simulink model "MDCC_DeadComp"  (R2023a)
settings: Solver=FixedStepDiscrete  StartTime=0.0  StopTime=10.0  FixedStep=0.0001  RelTol=1e-3
model workspace (MATLAB code in the model file):
  | cmdLim = Simulink.Parameter;
  | cmdLim.Value = 15;
  | cmdLim.Description = 'Limit for controlling the maximum surface command angle.';
  | cmdLim.Min = 0;
  | cmdLim.Max = 90;
  | cmdLim.DocUnits = 'deg';
  | 
  | dispGain = Simulink.Parameter;
  | dispGain.Value = 0.75;
  | dispGain.Description = 'Gain applied to the displacement error.';
  | dispGain.Min = 0;
  | dispGain.Max = [];
  | dispGain.DocUnits = 'deg/sec/deg';
  | 
  | dispLim = Simulink.Parameter;
  | dispLim.Value = 30;
  | dispLim.Description = 'Limit for controlling the maximum commanded angle.';
  | dispLim.Min = 0;
  | dispLim.Max = 180;
  | dispLim.DocUnits = 'deg';
  | 
  | intGain = Simulink.Parameter;
  | intGain.Value = 0.5;
  | intGain.Description = 'Gain applied to the integral error.';
  | intGain.Min = 0;
  | intGain.Max = [];
  | intGain.DocUnits = 'deg/sec/deg/sec';
  | 
  | intLim = Simulink.Parameter;
  | intLim.Value = 5;
  | intLim.Description = 'Limit for controlling the maximum commanded angle.';
  | intLim.Min = 0;
  | intLim.Max = 90;
  | intLim.DocUnits = 'deg';
  | 
  | rateGain = Simulink.Parameter;
  | rateGain.Value = 2;
  | rateGain.Description = 'Gain applied to the rate error.';
  | rateGain.Min = 0;
  | rateGain.Max = [];
  | rateGain.DocUnits = 'deg/deg/sec';
  | 
  | rateLim = Simulink.Parameter;
  | rateLim.Value = 6;
  | rateLim.Description = 'Limit for controlling the maximum commanded angle.';
  | rateLim.Min = 0;
  | rateLim.Max = 180;
  | rateLim.DocUnits = 'deg/sec';
  | 
  | hdgGain = Simulink.Parameter;
  | hdgGain.Value = 0.015;
values from neighbouring files (symbols this model uses):
  Ts = 5E-6    (= 5e-06)    [iPMSM_data.m]
undefined symbols (not defined in the file or in its folder): CosTable12bit_Y, GLBCal_GLBCal_Kf_DCLinkOverVolErrThd_V, GLBCal_GLBCal_Kf_DCLinkUnderVolErrThd_V, GLBCal_GLBCal_Kf_EquiLd_NULL, GLBCal_GLBCal_Kf_EquiLq_NULL, GLBCal_GLBCal_Kf_MotorRatedSpeed_rpm, GLBCal_GLBCal_Kf_MotorSpeedHysteresis_Coef, GLBCal_Ke_MotorPolePairsNum_NULL, IoHwAbOpArg_PwmDutyCyclePhU_NULL, IoHwAbOpArg_PwmDutyCyclePhV_NULL, IoHwAbOpArg_PwmDutyCyclePhW_NULL, IoHwAbOpArg_PwmOutputEn, KbMDCC_DeadTimeCompEn_flg, KbMDCC_MCF_flgHarmInject_flg, KbMDCC_SetEAngleEn_flg, KbMDCC_UdUqFwOmit_flg, KfMDCC_AbsIs_A, KfMDCC_ActiveDischargeIdCurVal_A, KfMDCC_ActiveDischargeIqCurVal_A, KfMDCC_DCLinkVolRate_coef, KfMDCC_DeadRate_NULL, KfMDCC_DebugEAngleInit_rad, KfMDCC_DebugUalphaVolCmd_V, KfMDCC_DebugUbetaVolCmd_V, KfMDCC_DebugUdCmd_V, KfMDCC_DebugUqCmd_V, KfMDCC_DebugUsCmd_V, KfMDCC_DebugUsRate_V, KfMDCC_Duty_Coef, KfMDCC_IMCResp_NULL, KfMDCC_IMCStab_NULL, KfMDCC_InvParkCpPeriodTimesT_NULL, KfMDCC_MCF_Harm1113FLParamSpeedThrd_rads, KfMDCC_MCF_Harm57FLParamSpeedThrd_rads, KfMDCC_MCF_HarmCpnAg_NULL, KfMDCC_MCF_HarmfLParaHigh_coef, KfMDCC_MCF_HarmfLParaLow_coef, KfMDCC_MCF_HarmInSpdLimt_rpm, KfMDCC_MCF_HarmInUAlphaMax_V, KfMDCC_MCF_HarmInUbetaMax_V, KfMDCC_MotorSpeedRadsDAQFactor_NULL, KfMDCC_ResScal_Coef, KfMDCC_SelfHeatingUdVal_V, KfMDCC_SelfHeatingUdValRate_V, KfMDCC_SpdIMCResp_rpm, KfMDCC_SpdIMCStab_rpm, KfMDCC_VfMDCC_DCLinkCurValFactor_NULL, KfMDCM_DCLinkCoef, KfMDCM_DCLinkRatedVoltage_V, KfMDCM_FluxWeakningVolFWOffset_V, KuMDCC_PositionResolution_NULL, KuMDCC_SetEAngle_Null, MDSM_MCUStatus, PiIoHwSetInvState_C_Sws_UVW_PwmEnOutput, PiIoHwSetInvState_C_SwsSet_DPO_UVW_Asc, PiIoHwSetInvState_C_SwsSet_DPO_UVW_FW, PiIoHwSetPwmDuty_C_SwsSet_DPO_UVW_Duty, SinTable12bit_Y, SVPWM, VfMDCC_DeadComSpeedHigh_Rpm ... (+5)
libraries: simulink x14, PMSM_Library x4
(part 3 of 6)

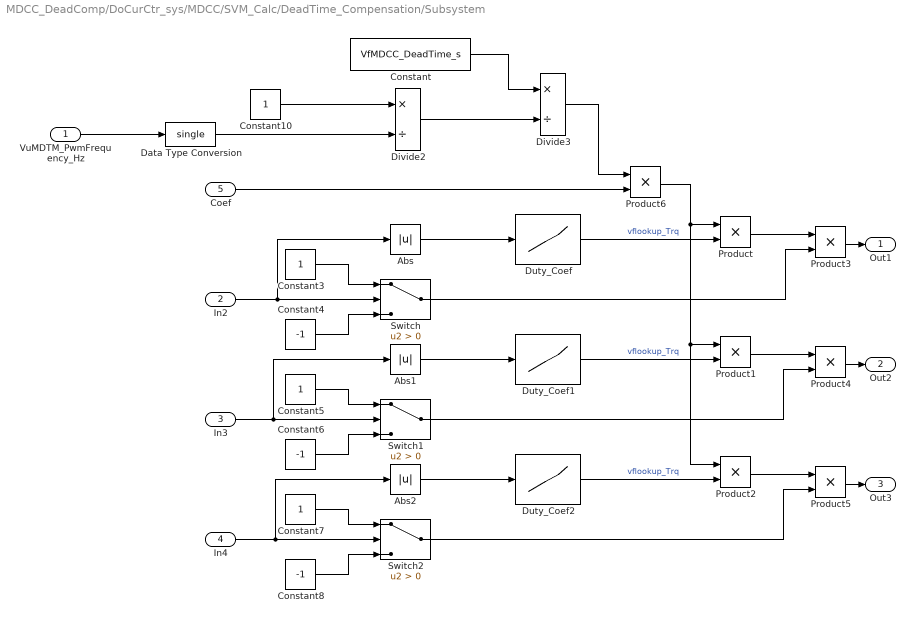
== system MDCC_DeadComp/DoCurCtr_sys/MDCC/SVM_Calc/DeadTime_Compensation/Subsystem ==
  VuMDTM_PwmFrequency_Hz : Inport
  In2 : Inport  Port=2
  In3 : Inport  Port=3
  In4 : Inport  Port=4
  Coef : Inport  Port=5
  Abs : Abs  SaturateOnIntegerOverflow=off
  Abs1 : Abs  SaturateOnIntegerOverflow=off
  Abs2 : Abs  SaturateOnIntegerOverflow=off
  Constant : Constant  Value=VfMDCC_DeadTime_s  OutDataTypeStr=single
  Constant10 : Constant  OutDataTypeStr=single
  Constant3 : Constant  OutDataTypeStr=int8
  Constant4 : Constant  Value=-1  OutDataTypeStr=int8
  Constant5 : Constant  OutDataTypeStr=int8
  Constant6 : Constant  Value=-1  OutDataTypeStr=int8
  Constant7 : Constant  OutDataTypeStr=int8
  Constant8 : Constant  Value=-1  OutDataTypeStr=int8
  Data Type Conversion : DataTypeConversion  OutDataTypeStr=single  SaturateOnIntegerOverflow=off  RndMeth=Floor
  Divide2 : Product  Inputs=*/
  Divide3 : Product  Inputs=*/
  Duty_Coef : Lookup_n-D  NumberOfTableDimensions=1  BreakpointsForDimension1=KfMDCC_AbsIs_A  BreakpointsForDimension1DataTypeStr=Inherit: Inherit from 'Breakpoint data'  IndexSearchMethod=Linear search  Table=KfMDCC_Duty_Coef  TableDataTypeStr=Inherit: Inherit from 'Table data'  ExtrapMethod=Clip  UseLastTableValue=on  InternalRulePriority=Speed  OutDataTypeStr=Inherit: Inherit from 'Table data'  RndMeth=Simplest  InputSameDT=off
  Duty_Coef1 : Lookup_n-D  NumberOfTableDimensions=1  BreakpointsForDimension1=KfMDCC_AbsIs_A  BreakpointsForDimension1DataTypeStr=Inherit: Inherit from 'Breakpoint data'  IndexSearchMethod=Linear search  Table=KfMDCC_Duty_Coef  TableDataTypeStr=Inherit: Inherit from 'Table data'  ExtrapMethod=Clip  UseLastTableValue=on  InternalRulePriority=Speed  OutDataTypeStr=Inherit: Inherit from 'Table data'  RndMeth=Simplest  InputSameDT=off
  Duty_Coef2 : Lookup_n-D  NumberOfTableDimensions=1  BreakpointsForDimension1=KfMDCC_AbsIs_A  BreakpointsForDimension1DataTypeStr=Inherit: Inherit from 'Breakpoint data'  IndexSearchMethod=Linear search  Table=KfMDCC_Duty_Coef  TableDataTypeStr=Inherit: Inherit from 'Table data'  ExtrapMethod=Clip  UseLastTableValue=on  InternalRulePriority=Speed  OutDataTypeStr=Inherit: Inherit from 'Table data'  RndMeth=Simplest  InputSameDT=off
  Product{,1..6} (7 alike) : Product
  Switch : Switch  Criteria=u2 > Threshold  SaturateOnIntegerOverflow=off  InputSameDT=off
  Switch1 : Switch  Criteria=u2 > Threshold  SaturateOnIntegerOverflow=off  InputSameDT=off
  Switch2 : Switch  Criteria=u2 > Threshold  SaturateOnIntegerOverflow=off  InputSameDT=off
  Out1 : Outport
  Out2 : Outport  Port=2
  Out3 : Outport  Port=3
  wires:
  Product/1 -> Product3/1
  Constant3/1 -> Switch/1
  Constant6/1 -> Switch1/3
  Constant8/1 -> Switch2/3
  Switch2/1 -> Product5/2
  Constant5/1 -> Switch1/1
  Duty_Coef1/1 -> Product1/2  "vflookup_Trq"
  Switch1/1 -> Product4/2
  Constant4/1 -> Switch/3
  Abs1/1 -> Duty_Coef1/1
  In4/1 -> Abs2/1, Switch2/2
  Product1/1 -> Product4/1
  Product2/1 -> Product5/1
  In3/1 -> Abs1/1, Switch1/2
  Constant7/1 -> Switch2/1
  Constant10/1 -> Divide2/1
  Abs2/1 -> Duty_Coef2/1
  Product5/1 -> Out3/1
  In2/1 -> Abs/1, Switch/2
  Duty_Coef2/1 -> Product2/2  "vflookup_Trq"
  Divide2/1 -> Divide3/2
  Duty_Coef/1 -> Product/2  "vflookup_Trq"
  Abs/1 -> Duty_Coef/1
  Constant/1 -> Divide3/1
  Switch/1 -> Product3/2
  Product3/1 -> Out1/1
  Product4/1 -> Out2/1
  VuMDTM_PwmFrequency_Hz/1 -> Data Type Conversion/1
  Data Type Conversion/1 -> Divide2/2
  Divide3/1 -> Product6/1
  Product6/1 -> Product2/1, Product1/1, Product/1
  Coef/1 -> Product6/2

== system MDCC_DeadComp/DoCurCtr_sys/MDCC/SVM_Calc/DeadTime_Compensation/TorqueDamping ==
  set : Inport
  Constant2 : Constant  Value=KfMDCC_DeadRate_NULL
  Delay : Delay  DelayLength=1
  Subsystem1 : Subsystem
  VfMDTL_TorqueCmd_Nm : Outport
  wires:
  Delay/1 -> Subsystem1/3(this_ref)
  Subsystem1/1(Out1) -> VfMDTL_TorqueCmd_Nm/1, Delay/1
  Constant2/1 -> Subsystem1/2(rate)
  set/1 -> Subsystem1/1(set)

== system MDCC_DeadComp/DoCurCtr_sys/MDCC/SVM_Calc/MDSA/SVPWM1 ==
  Ualpha_V : Inport
  Ubeta_V : Inport  Port=2
  Ts : Inport  Port=3
  Vdc : Inport  Port=4
  Bus Creator : BusCreator  Inputs=2
  Bus Creator1 : BusCreator  Inputs=2
  Bus Selector : BusSelector  OutputSignals=signal1,signal2,signal3
  Terminator : Terminator
  vIntp_PWMFOC_CalSec : Subsystem  TreatAsAtomicUnit=on  RTWFcnName=vIntp_PWMFOC_CalSec  RTWFileName=vIntp_PWMFOC_CalSec
      settings: RTWFcnNameOpts=User specified  RTWFileNameOpts=User specified
  vIntp_PWMFOC_CalTriCompValue : Subsystem  TreatAsAtomicUnit=on  RTWFcnName=vIntp_PWMFOC_CalTriCompValue  RTWFileName=vIntp_PWMFOC_CalTriCompValue
      settings: RTWFcnNameOpts=User specified  RTWFileNameOpts=User specified
  VfMDSA_PwmDutyCyclePhaseU_NULL : Outport
  VfMDSA_PwmDutyCyclePhaseV_NULL : Outport  Port=2
  VfMDSA_PwmDutyCyclePhaseW_NULL : Outport  Port=3
  wires:
  Bus Creator1/1 -> vIntp_PWMFOC_CalTriCompValue/3(Bus_Ts_Vdc)
  Vdc/1 -> Bus Creator1/2  "Vdc"
  Ts/1 -> Bus Creator1/1  "Ts"
  Ubeta_V/1 -> Bus Creator/2  "Ubeta"
  Ualpha_V/1 -> Bus Creator/1  "Ualpha"
  Bus Creator/1 -> vIntp_PWMFOC_CalSec/1(Bus_UalphaUbeta), vIntp_PWMFOC_CalTriCompValue/2(Bus_UalphaUbeta)
  vIntp_PWMFOC_CalSec/1(SecValue) -> Terminator/1
  vIntp_PWMFOC_CalSec/2(N_VALUE) -> vIntp_PWMFOC_CalTriCompValue/1(N_VALUE_IN)
  vIntp_PWMFOC_CalTriCompValue/1(Bus_CMP) -> Bus Selector/1
  Bus Selector/1 -> VfMDSA_PwmDutyCyclePhaseU_NULL/1  "<signal1>"
  Bus Selector/2 -> VfMDSA_PwmDutyCyclePhaseV_NULL/1  "<signal2>"
  Bus Selector/3 -> VfMDSA_PwmDutyCyclePhaseW_NULL/1  "<signal3>"

== system MDCC_DeadComp/DoCurCtr_sys/MDCC/SVM_Calc/MDSA/SVPWM_E ==
  Vsalfak : Inport
  Vsbetak : Inport  Port=2
  Udc : Inport  Port=3
  SVPWM1 : MATLAB Function  TreatAsAtomicUnit=on
  T1 : Outport
  T2 : Outport  Port=2
  T3 : Outport  Port=3
  wires:
  SVPWM1/1(T1) -> T1/1
  SVPWM1/2(T2) -> T2/1
  Vsalfak/1 -> SVPWM1/1(Vsalfak)
  Vsbetak/1 -> SVPWM1/2(Vsbetak)
  Udc/1 -> SVPWM1/3(Udc)
  SVPWM1/3(T3) -> T3/1

== system MDCC_DeadComp/DoCurCtr_sys/MDCC/Simulink Function/Subsystem/If Action Subsystem ==
  In1 : Inport
  Action Port : ActionPort  ActionPortLabel=if(u1 >= u2)
  Constant : Constant  Value=2*pi  OutDataTypeStr=single
  Subtract : Sum  Inputs=+-
  Out1 : Outport
  wires:
  In1/1 -> Subtract/1
  Constant/1 -> Subtract/2
  Subtract/1 -> Out1/1

== system MDCC_DeadComp/DoCurCtr_sys/MDCC/Simulink Function/Subsystem/If Action Subsystem1 ==
  In1 : Inport
  Action Port : ActionPort  ActionPortLabel=elseif(u1 <0)
  Constant : Constant  Value=2*pi  OutDataTypeStr=single
  Subtract : Sum
  Out1 : Outport
  wires:
  In1/1 -> Subtract/1
  Constant/1 -> Subtract/2
  Subtract/1 -> Out1/1

== system MDCC_DeadComp/DoCurCtr_sys/MDCC/Simulink Function/Subsystem/If Action Subsystem2 ==
  In1 : Inport
  Action Port : ActionPort  ActionPortLabel=else
  Out1 : Outport
  wires:
  In1/1 -> Out1/1

== system MDCC_DeadComp/DoCurCtr_sys/MDCC/UdUqCalc_Sys/MDCC_Inverse_Park_Transform/Do_Inverse_Park_Transform ==
  VfMDCC_UdVal_V : Inport
  VfMDCC_UqVal_V : Inport  Port=2
  VfMDCC_SinEAngleNextPWMValue_NULL : Inport  Port=3
  VfMDCC_CosEAngleNextPWMValue_NULL : Inport  Port=4
  Product{,1..3} (4 alike) : Product  RndMeth=Zero
  Subtract : Sum  Inputs=+-
  Subtract1 : Sum
  VfMDCC_VolCmd_alpha_V : Outport
  VfMDCC_VolCmd_beta_V : Outport  Port=2
  wires:
  VfMDCC_UdVal_V/1 -> Product2/1, Product/1
  Product3/1 -> Subtract1/2
  Product2/1 -> Subtract1/1
  Subtract1/1 -> VfMDCC_VolCmd_beta_V/1
  Subtract/1 -> VfMDCC_VolCmd_alpha_V/1
  Product1/1 -> Subtract/2
  VfMDCC_SinEAngleNextPWMValue_NULL/1 -> Product2/2, Product1/2
  VfMDCC_UqVal_V/1 -> Product1/1, Product3/1
  Product/1 -> Subtract/1
  VfMDCC_CosEAngleNextPWMValue_NULL/1 -> Product3/2, Product/2

== system MDCC_DeadComp/DoCurCtr_sys/MDCC/UdUqCalc_Sys/MDCC_MCF_Sys1/Clarke1 ==
  VfMDCC_PhaseUCurHarmonic_A : Inport
  VfMDCC_PhaseVCurHarmonic_A : Inport  Port=2
  VfMDCC_PhaseWCurHarmonic_A : Inport  Port=3
  Constant : Constant  Value=0.57735  OutDataTypeStr=single
  Data Type Conversion : DataTypeConversion  OutDataTypeStr=single  SaturateOnIntegerOverflow=off  RndMeth=Floor
  Product : Product
  Subtract : Sum  Inputs=+-
  VfMDCC_AlphaCurHarmonic_A : Outport
  VfMDCC_BetaCurHarmonic_A : Outport  Port=2
  wires:
  Data Type Conversion/1 -> VfMDCC_AlphaCurHarmonic_A/1  "VfMDCC_AlphaCurHarmonic_A"
  Product/1 -> VfMDCC_BetaCurHarmonic_A/1  "VfMDCC_BetaCurHarmonic_A"
  Constant/1 -> Product/2
  Subtract/1 -> Product/1
  VfMDCC_PhaseWCurHarmonic_A/1 -> Subtract/2
  VfMDCC_PhaseVCurHarmonic_A/1 -> Subtract/1
  VfMDCC_PhaseUCurHarmonic_A/1 -> Data Type Conversion/1

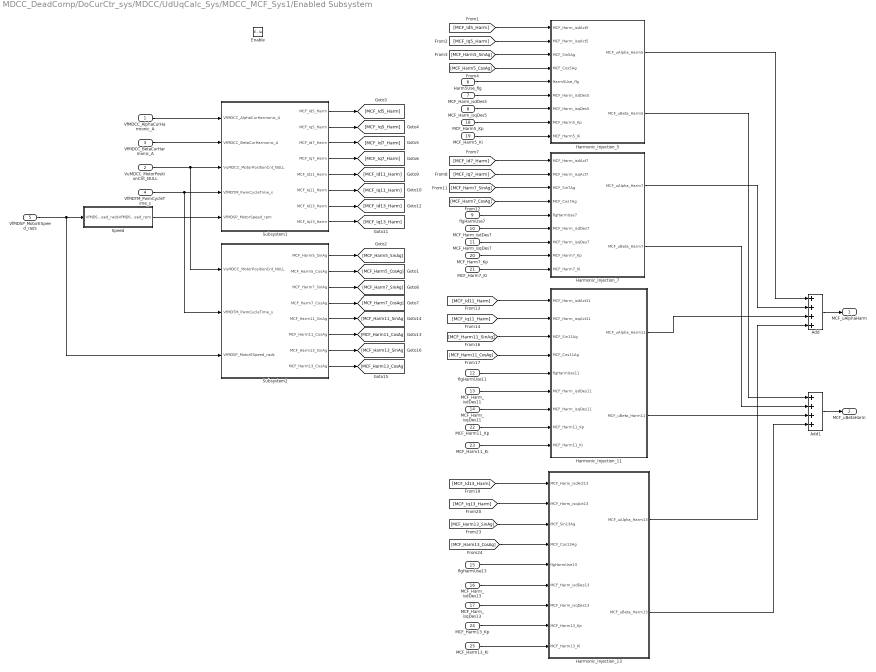
== system MDCC_DeadComp/DoCurCtr_sys/MDCC/UdUqCalc_Sys/MDCC_MCF_Sys1/Enabled Subsystem ==
  VfMDCC_AlphaCurHarmonic_A : Inport
  VuMDCC_MotorPositionCnt_NULL : Inport  Port=2
  VfMDCC_BetaCurHarmonic_A : Inport  Port=3
  VfMDTM_PwmCycleTime_s : Inport  Port=4
  VfMDSP_MotorESpeed_rads : Inport  Port=5
  Harm5Use_flg : Inport  Port=6
  MCF_Harm_isdDes5 : Inport  Port=7
  MCF_Harm_isqDes5 : Inport  Port=8
  flgHarmUse7 : Inport  Port=9
  MCF_Harm_isdDes7 : Inport  Port=10
  MCF_Harm_isqDes7 : Inport  Port=11
  flgHarmUse11 : Inport  Port=12
  MCF_Harm_isdDes11 : Inport  Port=13
  MCF_Harm_isqDes11 : Inport  Port=14
  flgHarmUse13 : Inport  Port=15
  MCF_Harm_isdDes13 : Inport  Port=16
  MCF_Harm_isqDes13 : Inport  Port=17
  MCF_Harm5_Kp : Inport  Port=18
  MCF_Harm5_Ki : Inport  Port=19
  MCF_Harm7_Kp : Inport  Port=20
  MCF_Harm7_Ki : Inport  Port=21
  MCF_Harm11_Kp : Inport  Port=22
  MCF_Harm11_Ki : Inport  Port=23
  MCF_Harm13_Kp : Inport  Port=24
  MCF_Harm13_Ki : Inport  Port=25
  Enable : EnablePort  StatesWhenEnabling=reset
  Add : Sum  Inputs=++++  OutDataTypeStr=single
  Add1 : Sum  Inputs=++++  AccumDataTypeStr=single
  Harmonic_Injection_11 : Subsystem
  Harmonic_Injection_13 : Subsystem
  Harmonic_Injection_5 : Subsystem
  Harmonic_Injection_7 : Subsystem
  Speed : Subsystem
  Subsystem1 : Subsystem
  Subsystem2 : Subsystem
  MCF_uAlphaHarm : Outport  VectorParamsAs1DForOutWhenUnconnected=off
  MCF_uBetaHarm : Outport  Port=2  VectorParamsAs1DForOutWhenUnconnected=off
  wires:
  VfMDCC_AlphaCurHarmonic_A/1 -> Subsystem1/1(VfMDCC_AlphaCurHarmonic_A)
  VuMDCC_MotorPositionCnt_NULL/1 -> Subsystem2/1(VuMDCC_MotorPositionCnt_NULL), Subsystem1/3(VuMDCC_MotorPositionCnt_NULL)
  VfMDCC_BetaCurHarmonic_A/1 -> Subsystem1/2(VfMDCC_BetaCurHarmonic_A)
  VfMDTM_PwmCycleTime_s/1 -> Subsystem2/2(VfMDTM_PwmCycleTime_s), Subsystem1/4(VfMDTM_PwmCycleTime_s)
  Subsystem1/1(MCF_Id5_Harm) -> [MCF_Id5_Harm]
  Subsystem1/2(MCF_Iq5_Harm) -> [MCF_Iq5_Harm]
  Subsystem1/3(MCF_Id7_Harm) -> [MCF_Id7_Harm]
  Subsystem1/4(MCF_Iq7_Harm) -> [MCF_Iq7_Harm]
  Subsystem1/5(MCF_Id11_Harm) -> [MCF_Id11_Harm]
  Subsystem1/6(MCF_Iq11_Harm) -> [MCF_Iq11_Harm]
  Subsystem1/7(MCF_Id13_Harm) -> [MCF_Id13_Harm]
  Subsystem1/8(MCF_Iq13_Harm) -> [MCF_Iq13_Harm]
  Subsystem2/1(MCF_Harm5_SinAg) -> [MCF_Harm5_SinAg]
  Subsystem2/2(MCF_Harm5_CosAg) -> [MCF_Harm5_CosAg]
  Subsystem2/3(MCF_Harm7_SinAg) -> [MCF_Harm7_SinAg]
  Subsystem2/4(MCF_Harm7_CosAg) -> [MCF_Harm7_CosAg]
  Subsystem2/5(MCF_Harm11_SinAg) -> [MCF_Harm11_SinAg]
  Subsystem2/6(MCF_Harm11_CosAg) -> [MCF_Harm11_CosAg]
  Subsystem2/7(MCF_Harm13_SinAg) -> [MCF_Harm13_SinAg]
  Subsystem2/8(MCF_Harm13_CosAg) -> [MCF_Harm13_CosAg]
  [MCF_Id5_Harm] -> Harmonic_Injection_5/1(MCF_Harm_isdAct5)
  [MCF_Iq5_Harm] -> Harmonic_Injection_5/2(MCF_Harm_isqAct5)
  [MCF_Harm5_SinAg] -> Harmonic_Injection_5/3(MCF_Sin5Ag)
  [MCF_Harm5_CosAg] -> Harmonic_Injection_5/4(MCF_Cos5Ag)
  [MCF_Id7_Harm] -> Harmonic_Injection_7/1(MCF_Harm_isdAct7)
  [MCF_Iq7_Harm] -> Harmonic_Injection_7/2(MCF_Harm_isqAct7)
  [MCF_Harm7_SinAg] -> Harmonic_Injection_7/3(MCF_Sin7Ag)
  [MCF_Harm7_CosAg] -> Harmonic_Injection_7/4(MCF_Cos7Ag)
  [MCF_Id11_Harm] -> Harmonic_Injection_11/1(MCF_Harm_isdAct11)
  [MCF_Iq11_Harm] -> Harmonic_Injection_11/2(MCF_Harm_isqAct11)
  [MCF_Harm11_SinAg] -> Harmonic_Injection_11/3(MCF_Sin11Ag)
  [MCF_Harm11_CosAg] -> Harmonic_Injection_11/4(MCF_Cos11Ag)
  [MCF_Id13_Harm] -> Harmonic_Injection_13/1(MCF_Harm_isdAct13)
  [MCF_Iq13_Harm] -> Harmonic_Injection_13/2(MCF_Harm_isqAct13)
  [MCF_Harm13_SinAg] -> Harmonic_Injection_13/3(MCF_Sin13Ag)
  [MCF_Harm13_CosAg] -> Harmonic_Injection_13/4(MCF_Cos13Ag)
  Add/1 -> MCF_uAlphaHarm/1
  Harmonic_Injection_5/2(MCF_uBeta_Harm5) -> Add1/1
  Harmonic_Injection_5/1(MCF_uAlpha_Harm5) -> Add/1
  Harmonic_Injection_11/2(MCF_uBeta_Harm11) -> Add1/3
  Add1/1 -> MCF_uBetaHarm/1
  Harmonic_Injection_13/1(MCF_uAlpha_Harm13) -> Add/4
  Harmonic_Injection_7/2(MCF_uBeta_Harm7) -> Add1/2
  Harmonic_Injection_11/1(MCF_uAlpha_Harm11) -> Add/3
  Harmonic_Injection_7/1(MCF_uAlpha_Harm7) -> Add/2
  Harmonic_Injection_13/2(MCF_uBeta_Harm13) -> Add1/4
  VfMDSP_MotorESpeed_rads/1 -> Speed/1(VfMDSP_MotorESpeed_rads), Subsystem2/3(VfMDSP_MotorESpeed_rads)
  Speed/1(VfMDSP_MotorAveSpeed_rpm) -> Subsystem1/5(VfMDSP_MotorSpeed_rpm)
  Harm5Use_flg/1 -> Harmonic_Injection_5/5(Harm5Use_flg)
  MCF_Harm_isdDes5/1 -> Harmonic_Injection_5/6(MCF_Harm_isdDes5)
  MCF_Harm_isqDes5/1 -> Harmonic_Injection_5/7(MCF_Harm_isqDes5)
  flgHarmUse7/1 -> Harmonic_Injection_7/5(flgHarmUse7)
  MCF_Harm_isdDes7/1 -> Harmonic_Injection_7/6(MCF_Harm_isdDes7)
  MCF_Harm_isqDes7/1 -> Harmonic_Injection_7/7(MCF_Harm_isqDes7)
  flgHarmUse11/1 -> Harmonic_Injection_11/5(flgHarmUse11)
  MCF_Harm_isdDes11/1 -> Harmonic_Injection_11/6(MCF_Harm_isdDes11)
  MCF_Harm_isqDes11/1 -> Harmonic_Injection_11/7(MCF_Harm_isqDes11)
  flgHarmUse13/1 -> Harmonic_Injection_13/5(flgHarmUse13)
  MCF_Harm_isdDes13/1 -> Harmonic_Injection_13/6(MCF_Harm_isdDes13)
  MCF_Harm_isqDes13/1 -> Harmonic_Injection_13/7(MCF_Harm_isqDes13)
  MCF_Harm5_Kp/1 -> Harmonic_Injection_5/8(MCF_Harm5_Kp)
  MCF_Harm5_Ki/1 -> Harmonic_Injection_5/9(MCF_Harm5_Ki)
  MCF_Harm7_Kp/1 -> Harmonic_Injection_7/8(MCF_Harm7_Kp)
  MCF_Harm7_Ki/1 -> Harmonic_Injection_7/9(MCF_Harm7_Ki)
  MCF_Harm11_Kp/1 -> Harmonic_Injection_11/8(MCF_Harm11_Kp)
  MCF_Harm11_Ki/1 -> Harmonic_Injection_11/9(MCF_Harm11_Ki)
  MCF_Harm13_Kp/1 -> Harmonic_Injection_13/8(MCF_Harm13_Kp)
  MCF_Harm13_Ki/1 -> Harmonic_Injection_13/9(MCF_Harm13_Ki)

== system MDCC_DeadComp/DoCurCtr_sys/MDCC/UdUqCalc_Sys/MDCC_MCF_Sys1/Subsystem ==
  VfMDSP_PhaseUCurVal_A : Inport  OutDataTypeStr=single
  VfMDSP_PhaseVCurVal_A : Inport  Port=2  OutDataTypeStr=single
  VfMDSP_PhaseWCurVal_A : Inport  Port=3  OutDataTypeStr=single
  VfMDTM_PwmCycleTime_s : Inport  Port=4  OutDataTypeStr=single
  VfMDSP_MotorESpeed_rads : Inport  Port=5  OutDataTypeStr=single
  Add : Sum  Inputs=+-
  Add1 : Sum  Inputs=+-
  Add2 : Sum  Inputs=+-
  Subsystem : Subsystem  TreatAsAtomicUnit=on
      settings: RTWSystemCode=Inline
  Subsystem1 : Subsystem  TreatAsAtomicUnit=on
      settings: RTWSystemCode=Inline
  Subsystem2 : Subsystem  TreatAsAtomicUnit=on
      settings: RTWSystemCode=Inline
  VfMDCC_PhaseUCurHarmonic_A : Outport
  VfMDCC_PhaseVCurHarmonic_A : Outport  Port=2
  VfMDCC_PhaseWCurHarmonic_A : Outport  Port=3
  wires:
  Subsystem2/1(Out1) -> Add2/2
  VfMDSP_PhaseUCurVal_A/1 -> Subsystem/1(VfMDSP_PhaseUCurVal_A), Add/1
  VfMDSP_MotorESpeed_rads/1 -> Subsystem2/2(VfMDSP_MotorESpeed_rads), Subsystem1/2(VfMDSP_MotorESpeed_rads), Subsystem/2(VfMDSP_MotorESpeed_rads)
  Subsystem/1(Out1) -> Add/2
  VfMDTM_PwmCycleTime_s/1 -> Subsystem2/3(VfMDTM_PwmCycleTime_s), Subsystem1/3(VfMDTM_PwmCycleTime_s), Subsystem/3(VfMDTM_PwmCycleTime_s)
  VfMDSP_PhaseVCurVal_A/1 -> Subsystem1/1(VfMDSP_PhaseUCurVal_A), Add1/1
  Add1/1 -> VfMDCC_PhaseVCurHarmonic_A/1  "VfMDCC_PhaseVCurHarmonic_A"
  VfMDSP_PhaseWCurVal_A/1 -> Subsystem2/1(VfMDSP_PhaseUCurVal_A), Add2/1
  Subsystem1/1(Out1) -> Add1/2
  Add/1 -> VfMDCC_PhaseUCurHarmonic_A/1  "VfMDCC_PhaseUCurHarmonic_A"
  Add2/1 -> VfMDCC_PhaseWCurHarmonic_A/1  "VfMDCC_PhaseWCurHarmonic_A"

== system MDCC_DeadComp/DoCurCtr_sys/MDCC/UdUqCalc_Sys/ModDegPwrFacCal/isCal ==
  id : Inport
  iq : Inport  Port=2
  Add : Sum
  Product : Product
  Product1 : Product
  Sqrt : Sqrt
  is : Outport
  wires:
  iq/1 -> Product1/2, Product1/1
  id/1 -> Product/2, Product/1
  Product1/1 -> Add/2
  Sqrt/1 -> is/1
  Product/1 -> Add/1
  Add/1 -> Sqrt/1

== system MDCC_DeadComp/DoCurCtr_sys/MDCC/UdUqCalc_Sys/ModDegPwrFacCal/pwrCal ==
  id : Inport
  iq : Inport  Port=2
  ud : Inport  Port=3
  uq : Inport  Port=4
  Add : Sum
  Product : Product
  Product1 : Product
  pwr : Outport
  wires:
  Product/1 -> Add/1  "IDUD"
  Product1/1 -> Add/2  "IQUQ"
  id/1 -> Product/1
  ud/1 -> Product/2
  iq/1 -> Product1/1
  uq/1 -> Product1/2
  Add/1 -> pwr/1

== system MDCC_DeadComp/DoCurCtr_sys/MDCC/UdUqCalc_Sys/ModDegPwrFacCal/usCal ==
  ud : Inport
  uq : Inport  Port=2
  Add : Sum
  Product : Product
  Product1 : Product
  Sqrt : Sqrt
  us : Outport
  wires:
  Add/1 -> Sqrt/1
  Product/1 -> Add/1
  Sqrt/1 -> us/1
  Product1/1 -> Add/2
  ud/1 -> Product/1, Product/2
  uq/1 -> Product1/1, Product1/2

== system MDCC_DeadComp/DoCurCtr_sys/MDCC/UdUqCalc_Sys/SelfHeating/Subsystem1 ==
  VfMDTM_SelfHeatingEAngle_NULL : Inport
  VbMDTM_SelfHeatingSinWaveEn_flg : Inport  Port=2
  VbMDSP_McuFSelfheatingMode_flg : Inport  Port=3
  Constant : Constant  Value=uint8(100)
  Constant1 : Constant  Value=KfMDCC_SelfHeatingUdVal_V
  Constant3 : Constant  Value=0  OutDataTypeStr=single
  Constant6 : Constant  Value=KfMDCC_SelfHeatingUdValRate_V
  Merge : Merge
  NOT : Logic  Operator=NOT  IconShape=distinctive  AllPortsSameDT=off  OutDataTypeStr=boolean
  Signal Copy : SignalConversion  OverrideOpt=off
  SinCounter_10ms : Subsystem  TreatAsAtomicUnit=on
      settings: RTWSystemCode=Nonreusable function  RTWFcnNameOpts=Use subsystem name
  Subsystem : Subsystem
  Subsystem1 : Subsystem
  Subsystem2 : Subsystem
  Switch : Switch  Criteria=u2 ~= 0  SaturateOnIntegerOverflow=off  InputSameDT=off
  VfMDCC_SelfHeatingUdVal_V : Outport
  VbMDCC_SelfHeatingStop_flg : Outport  Port=2
  wires:
  VfMDTM_SelfHeatingEAngle_NULL/1 -> Subsystem2/1(VfMDTM_SelfHeatingEAngle_NULL), Subsystem/1(VfMDTM_SelfHeatingEAngle_NULL)
  VbMDTM_SelfHeatingSinWaveEn_flg/1 -> NOT/1, Subsystem/Enable
  NOT/1 -> Subsystem2/Enable
  Subsystem/1(VfMDTM_SelfHeatingUdVal_V) -> Merge/1
  Subsystem2/1(VfMDTM_SelfHeatingUdVal_V) -> Merge/2
  Merge/1 -> Signal Copy/1  "MDCC_VfMDCC_SelfHeatingUdVal_V"
  Constant6/1 -> Subsystem1/2(rate)
  SinCounter_10ms/1(En) -> Subsystem1/Enable  "En"
  Constant/1 -> SinCounter_10ms/1(CNT)
  Subsystem1/1(VfMDTM_SelfHeatingUdVal_V_Set) -> Subsystem/2(VfMDTM_SelfHeatingUdVal_V_Set), Subsystem2/2(VfMDTM_SelfHeatingUdVal_V_Set)  "VfMDTM_SelfHeatingUdVal_V_Set"
  Subsystem1/2(VbMDCC_SelfHeatingStop_flg) -> VbMDCC_SelfHeatingStop_flg/1
  Constant3/1 -> Switch/3
  Constant1/1 -> Switch/1
  Switch/1 -> Subsystem1/1(set)
  VbMDSP_McuFSelfheatingMode_flg/1 -> Switch/2
  Signal Copy/1 -> VfMDCC_SelfHeatingUdVal_V/1

== system MDCC_DeadComp/DoCurCtr_sys/MDCC/UdUqCalc_Sys/UdUqCalc/IsDQCtl_200us ==
  PIReset : Inport
  TQC_IsdDes : Inport  Port=2
  TQC_IsqDes : Inport  Port=3
  ISM_Isd : Inport  Port=4
  ISM_Isq : Inport  Port=5
  TQC_omSttr : Inport  Port=6
  TQC_dtIsctl_Cc : Inport  Port=7
  TQC_kidq : Inport  Port=8
  TQC_kpd : Inport  Port=9
  TQC_kpq : Inport  Port=10
  TQC_Rv : Inport  Port=11
  TQC_UsqFluxExc : Inport  Port=12
  TQC_uDaMax_Cc : Inport  Port=13
  TQC_uQaMax_Cc : Inport  Port=14
  IsDQCtl_m : MATLAB Function  TreatAsAtomicUnit=on  VariantControl=IsDQCtl_m
      settings: RTWSystemCode=Nonreusable function  RTWFcnNameOpts=Use subsystem name
  TQC_UsdPI : Outport
  TQC_UsqPI : Outport  Port=2
  facIntglDa_Dbg : Outport  Port=3
  facIntglQa_Dbg : Outport  Port=4
  facIntglDaQa_Dbg : Outport  Port=5
  uDaUnlim_Dbg : Outport  Port=6
  uQaUnlim_Dbg : Outport  Port=7
  iDaDes_Dbg : Outport  Port=8
  iQaDes_Dbg : Outport  Port=9

== system MDCC_DeadComp/DoCurCtr_sys/MDCC/UdUqCalc_Sys/UdUqCalc/Subsystem ==
  VfMDSP_MotorAveAbsSpeed_rpm : Inport
  VfMDSP_MotorRs_Ohm : Inport  Port=2
  1-D Lookup Table : Lookup_n-D  NumberOfTableDimensions=1  BreakpointsForDimension1=KfMDCC_SpdIMCResp_rpm  BreakpointsForDimension1DataTypeStr=Inherit: Inherit from 'Breakpoint data'  IndexSearchMethod=Linear search  Table=KfMDCC_IMCResp_NULL  TableDataTypeStr=Inherit: Inherit from 'Table data'  ExtrapMethod=Clip  UseLastTableValue=on  InternalRulePriority=Speed  OutDataTypeStr=Inherit: Inherit from 'Table data'  RndMeth=Simplest  InputSameDT=off
  1-D Lookup Table1 : Lookup_n-D  NumberOfTableDimensions=1  BreakpointsForDimension1=KfMDCC_SpdIMCStab_rpm  BreakpointsForDimension1DataTypeStr=Inherit: Inherit from 'Breakpoint data'  IndexSearchMethod=Linear search  Table=KfMDCC_IMCStab_NULL  TableDataTypeStr=Inherit: Inherit from 'Table data'  ExtrapMethod=Clip  UseLastTableValue=on  InternalRulePriority=Speed  OutDataTypeStr=Inherit: Inherit from 'Table data'  RndMeth=Simplest  InputSameDT=off
  Add : Sum
  Constant : Constant  Value=GLBCal_GLBCal_Kf_EquiLq_NULL
  Constant1 : Constant  Value=GLBCal_GLBCal_Kf_EquiLd_NULL
  Product{,1,4..5} (4 alike) : Product  OutDataTypeStr=single  RndMeth=Round
  VfMDCC_Rv_Ohm : Outport
  KfMDCC_Kidq_NULL : Outport  Port=2
  KfMDCC_Kpd_NULL : Outport  Port=3
  KfMDCC_Kpq_NULL : Outport  Port=4
  wires:
  Product/1 -> VfMDCC_Rv_Ohm/1, Add/1  "VfMDCC_Rv_Ohm"
  VfMDSP_MotorAveAbsSpeed_rpm/1 -> 1-D Lookup Table/1, 1-D Lookup Table1/1
  Constant1/1 -> Product4/2
  [StabAdap] -> Product1/2
  1-D Lookup Table/1 -> [RespScal]  "VfMDCC_RespScal_NULL"
  1-D Lookup Table1/1 -> Product/1
  VfMDSP_MotorRs_Ohm/1 -> Product/2, Add/2
  [RespScal] -> Product4/1
  [RespScal] -> Product5/1
  [RespScal] -> Product1/1
  Constant/1 -> Product5/2
  Product1/1 -> KfMDCC_Kidq_NULL/1  "KfMDCC_Kidq_NULL"
  Add/1 -> [StabAdap]  "VfMDCC_KidqStabAdap_NULL"
  Product5/1 -> KfMDCC_Kpq_NULL/1  "KfMDCC_Kpq_NULL"
  Product4/1 -> KfMDCC_Kpd_NULL/1  "KfMDCC_Kpd_NULL"

== system MDCC_DeadComp/DoCurCtr_sys/MDCC/SVM_Calc/DeadTime_Compensation/TorqueDamping/Subsystem1 ==
  set : Inport
  rate : Inport  Port=2
  this_ref : Inport  Port=3
  Add : Sum  OutDataTypeStr=single
  Data Type Conversion : DataTypeConversion  OutDataTypeStr=single  SaturateOnIntegerOverflow=off  RndMeth=Floor
  MinMax : MinMax  Inputs=2  OutDataTypeStr=single
  MinMax1 : MinMax  Function=max  Inputs=2
  Subtract : Sum  Inputs=+-
  Out1 : Outport
  wires:
  rate/1 -> Subtract/2, Add/2
  MinMax1/1 -> Out1/1
  this_ref/1 -> Subtract/1, Add/1
  set/1 -> Data Type Conversion/1
  Add/1 -> MinMax/2
  Subtract/1 -> MinMax1/2
  MinMax/1 -> MinMax1/1
  Data Type Conversion/1 -> MinMax/1

== system MDCC_DeadComp/DoCurCtr_sys/MDCC/SVM_Calc/MDSA/SVPWM1/vIntp_PWMFOC_CalSec ==
  Bus_UalphaUbeta : Inport
  CalABC : Subsystem
  CalSecValue : Subsystem
  CalVaVbVc : Subsystem  TreatAsAtomicUnit=on
  SecValue : Outport
  N_VALUE : Outport  Port=2
  wires:
  CalVaVbVc/1(Bus_Vabc) -> CalABC/1(Bus_Vabc_IN)
  CalABC/1(Bus_ABC) -> CalSecValue/1(Bus_ABC_IN)
  CalSecValue/1(SecValue) -> SecValue/1
  Bus_UalphaUbeta/1 -> CalVaVbVc/1(Bus_UalphaUbeta)
  CalSecValue/2(N_VALUE) -> N_VALUE/1

== system MDCC_DeadComp/DoCurCtr_sys/MDCC/SVM_Calc/MDSA/SVPWM1/vIntp_PWMFOC_CalTriCompValue ==
  note: // 需要确定PWM的passive level
  N_VALUE_IN : Inport
  Bus_UalphaUbeta : Inport  Port=2
  Bus_Ts_Vdc : Inport  Port=3
  CalCMPValue : Subsystem
  CalTabc : Subsystem
  CalXYZ : Subsystem
  Bus_CMP : Outport
  wires:
  N_VALUE_IN/1 -> CalTabc/3(N_VALUE_IN), CalCMPValue/2(N_VALUE_IN)
  Bus_UalphaUbeta/1 -> CalXYZ/1(Bus_UalphaUbeta)
  CalXYZ/1(BUS_XYZ) -> CalTabc/1(Bus_XYZ_IN)
  CalTabc/1(Bus_Tabc) -> CalCMPValue/1(Bus_Tabc_IN)
  CalCMPValue/1(Bus_CMP) -> Bus_CMP/1
  Bus_Ts_Vdc/1 -> CalTabc/2(Bus_Ts_Vdc), CalXYZ/2(Bus_Ts_Vdc)

== system MDCC_DeadComp/DoCurCtr_sys/MDCC/UdUqCalc_Sys/MDCC_MCF_Sys1/Enabled Subsystem/Harmonic_Injection_11 ==
  MCF_Harm_isdAct11 : Inport
  MCF_Harm_isqAct11 : Inport  Port=2
  MCF_Sin11Ag : Inport  Port=3
  MCF_Cos11Ag : Inport  Port=4
  flgHarmUse11 : Inport  Port=5
  MCF_Harm_isdDes11 : Inport  Port=6
  MCF_Harm_isqDes11 : Inport  Port=7
  MCF_Harm11_Kp : Inport  Port=8
  MCF_Harm11_Ki : Inport  Port=9
  Bus Creator : BusCreator  Inputs=2
  Bus Creator1 : BusCreator  Inputs=2
  Bus Selector : BusSelector  OutputSignals=MCF_uAlpha_Harm11,MCF_uBeta_Harm11
  Signal Copy : SignalConversion  OverrideOpt=off
  Signal Copy1 : SignalConversion  OverrideOpt=off
  Subsystem : Subsystem
  Switch2 : Switch  Criteria=u2 ~= 0  SaturateOnIntegerOverflow=off  InputSameDT=off
  Unit Delay : UnitDelay  SampleTime=-1  HasFrameUpgradeWarning=on
  Zero : Constant  Value=0  OutDataTypeStr=single
  Zero1 : Constant  Value=0  OutDataTypeStr=single
  MCF_uAlpha_Harm11 : Outport
  MCF_uBeta_Harm11 : Outport  Port=2
  wires:
  Bus Selector/2 -> Signal Copy1/1  "<MCF_uBeta_Harm11>"
  Subsystem/1(MCF_uAlpha_Harm11) -> Bus Creator/1  "MCF_uAlpha_Harm11"
  Zero1/1 -> Bus Creator1/2  "MCF_uBeta_Harm11"
  Switch2/1 -> Bus Selector/1
  Bus Creator/1 -> Switch2/1
  Bus Creator1/1 -> Switch2/3
  Zero/1 -> Bus Creator1/1  "MCF_uAlpha_Harm11"
  Subsystem/2(MCF_uBeta_Harm11) -> Bus Creator/2  "MCF_uBeta_Harm11"
  Bus Selector/1 -> Signal Copy/1  "<MCF_uAlpha_Harm11>"
  flgHarmUse11/1 -> Subsystem/Enable, Switch2/2, Unit Delay/1  "flgHarmUse11"
  Signal Copy/1 -> MCF_uAlpha_Harm11/1  "VAR_MCF_uAlpha_Harm11_f32"
  Signal Copy1/1 -> MCF_uBeta_Harm11/1  "VAR_MCF_uBeta_Harm11_f32"
  MCF_Harm_isdAct11/1 -> Subsystem/3(MCF_Harm_isdAct11)
  MCF_Harm_isqAct11/1 -> Subsystem/4(MCF_Harm_isqAct11)
  Unit Delay/1 -> Subsystem/7(MCF_flgHarm11PIRest)
  MCF_Sin11Ag/1 -> Subsystem/5(MCF_Sin11Ag)
  MCF_Cos11Ag/1 -> Subsystem/6(MCF_Cos11Ag)
  MCF_Harm_isdDes11/1 -> Subsystem/1(MCF_Harm_isdDes11)
  MCF_Harm_isqDes11/1 -> Subsystem/2(MCF_Harm_isqDes11)
  MCF_Harm11_Kp/1 -> Subsystem/8(MCF_Harm11_Kp)
  MCF_Harm11_Ki/1 -> Subsystem/9(MCF_Harm11_Ki)

== system MDCC_DeadComp/DoCurCtr_sys/MDCC/UdUqCalc_Sys/MDCC_MCF_Sys1/Enabled Subsystem/Harmonic_Injection_13 ==
  MCF_Harm_isdAct13 : Inport
  MCF_Harm_isqAct13 : Inport  Port=2
  MCF_Sin13Ag : Inport  Port=3
  MCF_Cos13Ag : Inport  Port=4
  flgHarmUse13 : Inport  Port=5
  MCF_Harm_isdDes13 : Inport  Port=6
  MCF_Harm_isqDes13 : Inport  Port=7
  MCF_Harm13_Kp : Inport  Port=8
  MCF_Harm13_Ki : Inport  Port=9
  Bus Creator : BusCreator  Inputs=2
  Bus Creator1 : BusCreator  Inputs=2
  Bus Selector : BusSelector  OutputSignals=MCF_uAlpha_Harm13,MCF_uBeta_Harm13
  Signal Copy : SignalConversion  OverrideOpt=off
  Signal Copy1 : SignalConversion  OverrideOpt=off
  Subsystem : Subsystem
  Switch2 : Switch  Criteria=u2 ~= 0  SaturateOnIntegerOverflow=off  InputSameDT=off
  Unit Delay : UnitDelay  SampleTime=-1  HasFrameUpgradeWarning=on
  Zero : Constant  Value=0  OutDataTypeStr=single
  Zero1 : Constant  Value=0  OutDataTypeStr=single
  MCF_uAlpha_Harm13 : Outport
  MCF_uBeta_Harm13 : Outport  Port=2
  wires:
  Bus Selector/2 -> Signal Copy1/1  "<MCF_uBeta_Harm13>"
  Subsystem/1(MCF_uAlpha_Harm13) -> Bus Creator/1  "MCF_uAlpha_Harm13"
  Zero1/1 -> Bus Creator1/2  "MCF_uBeta_Harm13"
  Switch2/1 -> Bus Selector/1
  Bus Creator/1 -> Switch2/1
  Bus Creator1/1 -> Switch2/3
  Zero/1 -> Bus Creator1/1  "MCF_uAlpha_Harm13"
  Subsystem/2(MCF_uBeta_Harm13) -> Bus Creator/2  "MCF_uBeta_Harm13"
  Bus Selector/1 -> Signal Copy/1  "<MCF_uAlpha_Harm13>"
  flgHarmUse13/1 -> Unit Delay/1, Switch2/2, Subsystem/Enable  "flgHarmUse13"
  Signal Copy/1 -> MCF_uAlpha_Harm13/1  "VAR_MCF_uAlpha_Harm13_f32"
  Signal Copy1/1 -> MCF_uBeta_Harm13/1  "VAR_MCF_uBeta_Harm13_f32"
  MCF_Harm_isdAct13/1 -> Subsystem/3(MCF_Harm_isdAct13)
  MCF_Harm_isqAct13/1 -> Subsystem/4(MCF_Harm_isqAct13)
  Unit Delay/1 -> Subsystem/7(MCF_flgHarm13PIRest)
  MCF_Sin13Ag/1 -> Subsystem/5(MCF_Sin13Ag)
  MCF_Cos13Ag/1 -> Subsystem/6(MCF_Cos13Ag)
  MCF_Harm_isdDes13/1 -> Subsystem/1(MCF_Harm_isdDes13)
  MCF_Harm_isqDes13/1 -> Subsystem/2(MCF_Harm_isqDes13)
  MCF_Harm13_Kp/1 -> Subsystem/8(MCF_Harm13_Kp)
  MCF_Harm13_Ki/1 -> Subsystem/9(MCF_Harm13_Ki)

== system MDCC_DeadComp/DoCurCtr_sys/MDCC/UdUqCalc_Sys/MDCC_MCF_Sys1/Enabled Subsystem/Harmonic_Injection_5 ==
  MCF_Harm_isdAct5 : Inport
  MCF_Harm_isqAct5 : Inport  Port=2
  MCF_Sin5Ag : Inport  Port=3
  MCF_Cos5Ag : Inport  Port=4
  Harm5Use_flg : Inport  Port=5
  MCF_Harm_isdDes5 : Inport  Port=6
  MCF_Harm_isqDes5 : Inport  Port=7
  MCF_Harm5_Kp : Inport  Port=8
  MCF_Harm5_Ki : Inport  Port=9
  Bus Creator : BusCreator  Inputs=2
  Bus Creator1 : BusCreator  Inputs=2
  Bus Selector : BusSelector  OutputSignals=MCF_uAlpha_Harm5,MCF_uBeta_Harm5
  Signal Copy : SignalConversion  OverrideOpt=off
  Signal Copy1 : SignalConversion  OverrideOpt=off
  Subsystem : Subsystem
  Switch2 : Switch  Criteria=u2 ~= 0  SaturateOnIntegerOverflow=off  InputSameDT=off
  Unit Delay : UnitDelay  SampleTime=-1  HasFrameUpgradeWarning=on
  Zero : Constant  Value=0  OutDataTypeStr=single
  Zero1 : Constant  Value=0  OutDataTypeStr=single
  MCF_uAlpha_Harm5 : Outport
  MCF_uBeta_Harm5 : Outport  Port=2
  wires:
  Bus Selector/2 -> Signal Copy1/1  "<MCF_uBeta_Harm5>"
  Subsystem/1(MCF_uAlpha_Harm5) -> Bus Creator/1  "MCF_uAlpha_Harm5"
  Zero1/1 -> Bus Creator1/2  "MCF_uBeta_Harm5"
  Switch2/1 -> Bus Selector/1
  Bus Creator/1 -> Switch2/1
  Bus Creator1/1 -> Switch2/3
  Zero/1 -> Bus Creator1/1  "MCF_uAlpha_Harm5"
  Subsystem/2(MCF_uBeta_Harm5) -> Bus Creator/2  "MCF_uBeta_Harm5"
  Bus Selector/1 -> Signal Copy/1  "<MCF_uAlpha_Harm5>"
  Harm5Use_flg/1 -> Subsystem/Enable, Switch2/2, Unit Delay/1  "flgHarmUse5"
  Signal Copy/1 -> MCF_uAlpha_Harm5/1  "VAR_MCF_uAlpha_Harm5_f32"
  Signal Copy1/1 -> MCF_uBeta_Harm5/1  "VAR_MCF_uBeta_Harm5_f32"
  MCF_Harm_isdAct5/1 -> Subsystem/3(MCF_Harm_isdAct5)
  MCF_Harm_isqAct5/1 -> Subsystem/4(MCF_Harm_isqAct5)
  Unit Delay/1 -> Subsystem/7(MCF_flgHarm5PIRest)
  MCF_Sin5Ag/1 -> Subsystem/5(MCF_Sin5Ag)
  MCF_Cos5Ag/1 -> Subsystem/6(MCF_Cos5Ag)
  MCF_Harm_isdDes5/1 -> Subsystem/1(MCF_Harm_isdDes5)
  MCF_Harm_isqDes5/1 -> Subsystem/2(MCF_Harm_isqDes5)
  MCF_Harm5_Kp/1 -> Subsystem/8(MCF_Harm5_Kp)
  MCF_Harm5_Ki/1 -> Subsystem/9(MCF_Harm5_Ki)

== system MDCC_DeadComp/DoCurCtr_sys/MDCC/UdUqCalc_Sys/MDCC_MCF_Sys1/Enabled Subsystem/Harmonic_Injection_7 ==
  MCF_Harm_isdAct7 : Inport
  MCF_Harm_isqAct7 : Inport  Port=2
  MCF_Sin7Ag : Inport  Port=3
  MCF_Cos7Ag : Inport  Port=4
  flgHarmUse7 : Inport  Port=5
  MCF_Harm_isdDes7 : Inport  Port=6
  MCF_Harm_isqDes7 : Inport  Port=7
  MCF_Harm7_Kp : Inport  Port=8
  MCF_Harm7_Ki : Inport  Port=9
  Bus Creator : BusCreator  Inputs=2
  Bus Creator1 : BusCreator  Inputs=2
  Bus Selector : BusSelector  OutputSignals=MCF_uAlpha_Harm7,MCF_uBeta_Harm7
  Signal Copy : SignalConversion  OverrideOpt=off
  Signal Copy1 : SignalConversion  OverrideOpt=off
  Subsystem : Subsystem
  Switch2 : Switch  Criteria=u2 ~= 0  SaturateOnIntegerOverflow=off  InputSameDT=off
  Unit Delay : UnitDelay  SampleTime=-1  HasFrameUpgradeWarning=on
  Zero : Constant  Value=0  OutDataTypeStr=single
  Zero1 : Constant  Value=0  OutDataTypeStr=single
  MCF_uAlpha_Harm7 : Outport
  MCF_uBeta_Harm7 : Outport  Port=2
  wires:
  Bus Selector/2 -> Signal Copy1/1  "<MCF_uBeta_Harm7>"
  Subsystem/1(MCF_uAlpha_Harm7) -> Bus Creator/1  "MCF_uAlpha_Harm7"
  Zero1/1 -> Bus Creator1/2  "MCF_uBeta_Harm7"
  Switch2/1 -> Bus Selector/1
  Bus Creator/1 -> Switch2/1
  Bus Creator1/1 -> Switch2/3
  Zero/1 -> Bus Creator1/1  "MCF_uAlpha_Harm7"
  Subsystem/2(MCF_uBeta_Harm7) -> Bus Creator/2  "MCF_uBeta_Harm7"
  Bus Selector/1 -> Signal Copy/1  "<MCF_uAlpha_Harm7>"
  flgHarmUse7/1 -> Subsystem/Enable, Switch2/2, Unit Delay/1  "flgHarmUse7"
  Signal Copy/1 -> MCF_uAlpha_Harm7/1  "VAR_MCF_uAlpha_Harm7_f32"
  Signal Copy1/1 -> MCF_uBeta_Harm7/1  "VAR_MCF_uBeta_Harm7_f32"
  MCF_Harm_isdAct7/1 -> Subsystem/3(MCF_Harm_isdAct7)
  MCF_Harm_isqAct7/1 -> Subsystem/4(MCF_Harm_isqAct7)
  Unit Delay/1 -> Subsystem/7(MCF_flgHarm7PIRest)
  MCF_Sin7Ag/1 -> Subsystem/5(MCF_Sin7Ag)
  MCF_Cos7Ag/1 -> Subsystem/6(MCF_Cos7Ag)
  MCF_Harm_isdDes7/1 -> Subsystem/1(MCF_Harm_isdDes7)
  MCF_Harm_isqDes7/1 -> Subsystem/2(MCF_Harm_isqDes7)
  MCF_Harm7_Kp/1 -> Subsystem/8(MCF_Harm7_Kp)
  MCF_Harm7_Ki/1 -> Subsystem/9(MCF_Harm7_Ki)

== system MDCC_DeadComp/DoCurCtr_sys/MDCC/UdUqCalc_Sys/MDCC_MCF_Sys1/Enabled Subsystem/Speed ==
  VfMDSP_MotorESpeed_rads : Inport
  Divide : Product  Inputs=*/
  GLBCal_Ke_MotorPolePairsNum_NULL : Constant  Value=GLBCal_Ke_MotorPolePairsNum_NULL
  Gain : Gain  Gain=single(30/pi)
  VfMDSP_MotorAveSpeed_rpm : Outport
  wires:
  VfMDSP_MotorESpeed_rads/1 -> Divide/1
  GLBCal_Ke_MotorPolePairsNum_NULL/1 -> Divide/2
  Divide/1 -> Gain/1
  Gain/1 -> VfMDSP_MotorAveSpeed_rpm/1

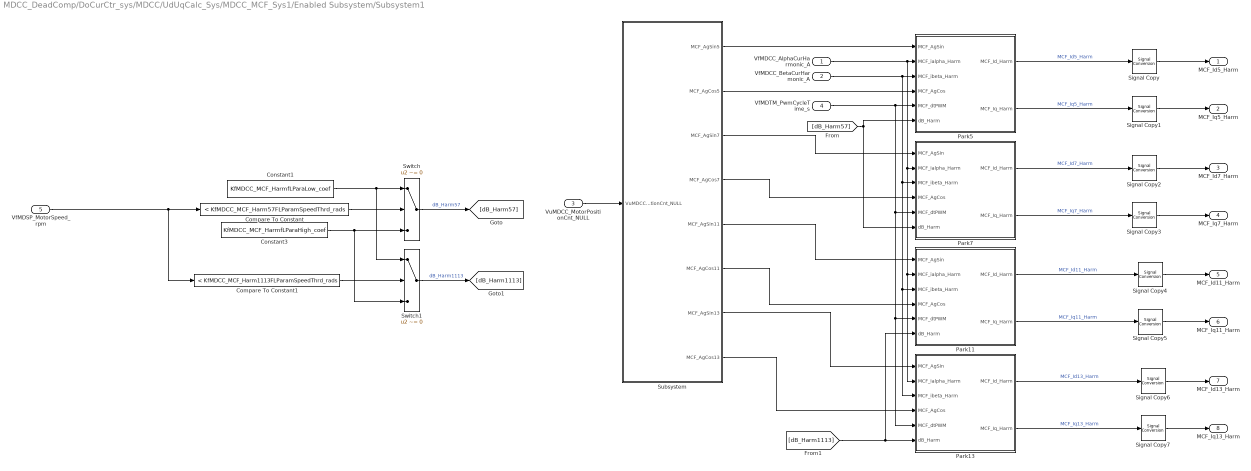
== system MDCC_DeadComp/DoCurCtr_sys/MDCC/UdUqCalc_Sys/MDCC_MCF_Sys1/Enabled Subsystem/Subsystem1 ==
  VfMDCC_AlphaCurHarmonic_A : Inport
  VfMDCC_BetaCurHarmonic_A : Inport  Port=2
  VuMDCC_MotorPositionCnt_NULL : Inport  Port=3
  VfMDTM_PwmCycleTime_s : Inport  Port=4
  VfMDSP_MotorSpeed_rpm : Inport  Port=5
  Compare To Constant : simulink/Logic and Bit Operations/Compare To Constant  relop=<  const=KfMDCC_MCF_Harm57FLParamSpeedThrd_rads  OutDataTypeStr=boolean
  Compare To Constant1 : simulink/Logic and Bit Operations/Compare To Constant  relop=<  const=KfMDCC_MCF_Harm1113FLParamSpeedThrd_rads  OutDataTypeStr=boolean
  Constant1 : Constant  Value=KfMDCC_MCF_HarmfLParaLow_coef  OutDataTypeStr=single
  Constant3 : Constant  Value=KfMDCC_MCF_HarmfLParaHigh_coef  OutDataTypeStr=single
  Park11 : Subsystem  TreatAsAtomicUnit=on  RTWFcnName=Harm_Park_Calc
      settings: RTWFcnNameOpts=User specified
  Park13 : Subsystem  TreatAsAtomicUnit=on  RTWFcnName=Harm_Park_Calc
      settings: RTWFcnNameOpts=User specified
  Park5 : Subsystem  TreatAsAtomicUnit=on  RTWFcnName=Harm_Park_Calc
      settings: RTWFcnNameOpts=User specified
  Park7 : Subsystem  TreatAsAtomicUnit=on  RTWFcnName=Harm_Park_Calc
      settings: RTWFcnNameOpts=User specified
  Signal Copy{,1..7} (8 alike) : SignalConversion  OverrideOpt=off
  Subsystem : Subsystem
  Switch : Switch  Criteria=u2 ~= 0  SaturateOnIntegerOverflow=off  InputSameDT=off
  Switch1 : Switch  Criteria=u2 ~= 0  SaturateOnIntegerOverflow=off  InputSameDT=off
  MCF_Id5_Harm : Outport
  MCF_Iq5_Harm : Outport  Port=2
  MCF_Id7_Harm : Outport  Port=3
  MCF_Iq7_Harm : Outport  Port=4
  MCF_Id11_Harm : Outport  Port=5
  MCF_Iq11_Harm : Outport  Port=6
  MCF_Id13_Harm : Outport  Port=7
  MCF_Iq13_Harm : Outport  Port=8
  wires:
  Subsystem/5(MCF_AgSin11) -> Park11/1(MCF_AgSin)
  VfMDCC_AlphaCurHarmonic_A/1 -> Park13/2(MCF_ialpha_Harm), Park11/2(MCF_ialpha_Harm), Park7/2(MCF_ialpha_Harm), Park5/2(MCF_ialpha_Harm)
  Constant1/1 -> Switch/1, Switch1/1
  [dB_Harm1113] -> Park11/6(dB_Harm), Park13/6(dB_Harm)
  Switch1/1 -> [dB_Harm1113]  "dB_Harm1113"
  Subsystem/8(MCF_AgCos13) -> Park13/4(MCF_AgCos)
  VuMDCC_MotorPositionCnt_NULL/1 -> Subsystem/1(VuMDCC_MotorPositionCnt_NULL)
  VfMDTM_PwmCycleTime_s/1 -> Park13/5(MCF_dtPWM), Park11/5(MCF_dtPWM), Park7/5(MCF_dtPWM), Park5/5(MCF_dtPWM)
  Subsystem/4(MCF_AgCos7) -> Park7/4(MCF_AgCos)
  Compare To Constant1/1 -> Switch1/2
  Subsystem/3(MCF_AgSin7) -> Park7/1(MCF_AgSin)
  VfMDSP_MotorSpeed_rpm/1 -> Compare To Constant/1, Compare To Constant1/1
  VfMDCC_BetaCurHarmonic_A/1 -> Park13/3(MCF_ibeta_Harm), Park11/3(MCF_ibeta_Harm), Park7/3(MCF_ibeta_Harm), Park5/3(MCF_ibeta_Harm)
  Switch/1 -> [dB_Harm57]  "dB_Harm57"
  Subsystem/2(MCF_AgCos5) -> Park5/4(MCF_AgCos)
  Compare To Constant/1 -> Switch/2
  Subsystem/7(MCF_AgSin13) -> Park13/1(MCF_AgSin)
  [dB_Harm57] -> Park5/6(dB_Harm), Park7/6(dB_Harm)
  Subsystem/1(MCF_AgSin5) -> Park5/1(MCF_AgSin)
  Subsystem/6(MCF_AgCos11) -> Park11/4(MCF_AgCos)
  Constant3/1 -> Switch1/3, Switch/3
  Signal Copy/1 -> MCF_Id5_Harm/1
  Park5/1(MCF_Id_Harm) -> Signal Copy/1  "MCF_Id5_Harm"
  Park5/2(MCF_Iq_Harm) -> Signal Copy1/1  "MCF_Iq5_Harm"
  Signal Copy1/1 -> MCF_Iq5_Harm/1
  Park7/1(MCF_Id_Harm) -> Signal Copy2/1  "MCF_Id7_Harm"
  Park7/2(MCF_Iq_Harm) -> Signal Copy3/1  "MCF_Iq7_Harm"
  Park11/1(MCF_Id_Harm) -> Signal Copy4/1  "MCF_Id11_Harm"
  Park11/2(MCF_Iq_Harm) -> Signal Copy5/1  "MCF_Iq11_Harm"
  Park13/1(MCF_Id_Harm) -> Signal Copy6/1  "MCF_Id13_Harm"
  Park13/2(MCF_Iq_Harm) -> Signal Copy7/1  "MCF_Iq13_Harm"
  Signal Copy2/1 -> MCF_Id7_Harm/1
  Signal Copy3/1 -> MCF_Iq7_Harm/1
  Signal Copy4/1 -> MCF_Id11_Harm/1
  Signal Copy5/1 -> MCF_Iq11_Harm/1
  Signal Copy6/1 -> MCF_Id13_Harm/1
  Signal Copy7/1 -> MCF_Iq13_Harm/1

== system MDCC_DeadComp/DoCurCtr_sys/MDCC/UdUqCalc_Sys/MDCC_MCF_Sys1/Enabled Subsystem/Subsystem2 ==
  VuMDCC_MotorPositionCnt_NULL : Inport
  VfMDTM_PwmCycleTime_s : Inport  Port=2
  VfMDSP_MotorESpeed_rads : Inport  Port=3
  Constant1 : Constant  Value=7  OutDataTypeStr=single
  Constant2 : Constant  Value=-5  OutDataTypeStr=single
  Constant3 : Constant  Value=-11  OutDataTypeStr=single
  Constant4 : Constant  Value=13  OutDataTypeStr=single
  Mcf_AgTranCalc1 : Subsystem
  Mcf_AgTranCalc2 : Subsystem
  Mcf_AgTranCalc3 : Subsystem
  Mcf_AgTranCalc5 : Subsystem
  Subsystem : Subsystem
  MCF_Harm5_SinAg : Outport
  MCF_Harm5_CosAg : Outport  Port=2
  MCF_Harm7_SinAg : Outport  Port=3
  MCF_Harm7_CosAg : Outport  Port=4
  MCF_Harm11_SinAg : Outport  Port=5
  MCF_Harm11_CosAg : Outport  Port=6
  MCF_Harm13_SinAg : Outport  Port=7
  MCF_Harm13_CosAg : Outport  Port=8
  wires:
  Mcf_AgTranCalc5/1(MCF_SinAg) -> MCF_Harm5_SinAg/1  "MCF_Harm5_SinAg"
  Mcf_AgTranCalc5/2(MCF_CosAg) -> MCF_Harm5_CosAg/1  "MCF_Harm5_CosAg"
  Mcf_AgTranCalc1/2(MCF_CosAg) -> MCF_Harm7_CosAg/1  "MCF_Harm7_CosAg"
  Mcf_AgTranCalc1/1(MCF_SinAg) -> MCF_Harm7_SinAg/1  "MCF_Harm7_SinAg"
  Mcf_AgTranCalc2/1(MCF_SinAg) -> MCF_Harm11_SinAg/1  "MCF_Harm11_SinAg"
  Mcf_AgTranCalc2/2(MCF_CosAg) -> MCF_Harm11_CosAg/1  "MCF_Harm11_CosAg"
  Mcf_AgTranCalc3/1(MCF_SinAg) -> MCF_Harm13_SinAg/1  "MCF_Harm13_SinAg"
  Mcf_AgTranCalc3/2(MCF_CosAg) -> MCF_Harm13_CosAg/1  "MCF_Harm13_CosAg"
  VfMDTM_PwmCycleTime_s/1 -> Subsystem/2(dtPwmWoRpwm)
  VfMDSP_MotorESpeed_rads/1 -> Subsystem/1(HSPF_nSlowFlt)
  Subsystem/1(Harm_AgCpn) -> Mcf_AgTranCalc1/1(Harm_AgCpn), Mcf_AgTranCalc3/1(Harm_AgCpn), Mcf_AgTranCalc2/1(Harm_AgCpn), Mcf_AgTranCalc5/1(Harm_AgCpn)
  VuMDCC_MotorPositionCnt_NULL/1 -> Subsystem/3(MCF_agRtrEe)
  Constant2/1 -> Mcf_AgTranCalc5/2(Harm_coef)
  Constant1/1 -> Mcf_AgTranCalc1/2(Harm_coef)
  Constant3/1 -> Mcf_AgTranCalc2/2(Harm_coef)
  Constant4/1 -> Mcf_AgTranCalc3/2(Harm_coef)

== system MDCC_DeadComp/DoCurCtr_sys/MDCC/UdUqCalc_Sys/MDCC_MCF_Sys1/Subsystem/Subsystem ==
  VfMDSP_PhaseUCurVal_A : Inport
  VfMDSP_MotorESpeed_rads : Inport  Port=2
  VfMDTM_PwmCycleTime_s : Inport  Port=3
  Add3 : Sum  Inputs=-+
  Add4 : Sum  Inputs=+-
  Add5 : Sum
  Add6 : Sum
  Divide : Product  Inputs=**
  Divide1 : Product  Inputs=**
  Divide2 : Product  Inputs=**
  Gain : Gain  Gain=1.414
  Unit Delay : UnitDelay  SampleTime=-1  HasFrameUpgradeWarning=on
  Unit Delay1 : UnitDelay  SampleTime=-1  HasFrameUpgradeWarning=on
  Unit Delay2 : UnitDelay  SampleTime=-1  HasFrameUpgradeWarning=on
  Out1 : Outport
  wires:
  Divide/1 -> Add5/2
  Unit Delay2/1 -> Add6/1, Add4/2
  Divide2/1 -> Divide1/1, Divide/2
  Add4/1 -> Divide/1
  Unit Delay1/1 -> Add5/1, Add3/1
  Unit Delay/1 -> Add3/2
  Add5/1 -> Out1/1, Divide1/2, Unit Delay1/1
  Add6/1 -> Unit Delay2/1
  Add3/1 -> Gain/1
  Gain/1 -> Add4/1
  Divide1/1 -> Add6/2
  VfMDSP_MotorESpeed_rads/1 -> Divide2/1
  VfMDTM_PwmCycleTime_s/1 -> Divide2/2
  VfMDSP_PhaseUCurVal_A/1 -> Unit Delay/1

== system MDCC_DeadComp/DoCurCtr_sys/MDCC/UdUqCalc_Sys/MDCC_MCF_Sys1/Subsystem/Subsystem1 ==
  VfMDSP_PhaseUCurVal_A : Inport
  VfMDSP_MotorESpeed_rads : Inport  Port=2
  VfMDTM_PwmCycleTime_s : Inport  Port=3
  Add3 : Sum  Inputs=-+
  Add4 : Sum  Inputs=+-
  Add5 : Sum
  Add6 : Sum
  Divide : Product  Inputs=**
  Divide1 : Product  Inputs=**
  Divide2 : Product  Inputs=**
  Gain : Gain  Gain=1.414
  Unit Delay : UnitDelay  SampleTime=-1  HasFrameUpgradeWarning=on
  Unit Delay1 : UnitDelay  SampleTime=-1  HasFrameUpgradeWarning=on
  Unit Delay2 : UnitDelay  SampleTime=-1  HasFrameUpgradeWarning=on
  Out1 : Outport
  wires:
  VfMDSP_PhaseUCurVal_A/1 -> Unit Delay/1
  VfMDTM_PwmCycleTime_s/1 -> Divide2/2
  VfMDSP_MotorESpeed_rads/1 -> Divide2/1
  Divide1/1 -> Add6/2
  Gain/1 -> Add4/1
  Add3/1 -> Gain/1
  Add6/1 -> Unit Delay2/1
  Add5/1 -> Unit Delay1/1, Divide1/2, Out1/1
  Unit Delay/1 -> Add3/2
  Unit Delay1/1 -> Add3/1, Add5/1
  Add4/1 -> Divide/1
  Divide2/1 -> Divide/2, Divide1/1
  Unit Delay2/1 -> Add4/2, Add6/1
  Divide/1 -> Add5/2

== system MDCC_DeadComp/DoCurCtr_sys/MDCC/UdUqCalc_Sys/MDCC_MCF_Sys1/Subsystem/Subsystem2 ==
  VfMDSP_PhaseUCurVal_A : Inport
  VfMDSP_MotorESpeed_rads : Inport  Port=2
  VfMDTM_PwmCycleTime_s : Inport  Port=3
  Add3 : Sum  Inputs=-+
  Add4 : Sum  Inputs=+-
  Add5 : Sum
  Add6 : Sum
  Divide : Product  Inputs=**
  Divide1 : Product  Inputs=**
  Divide2 : Product  Inputs=**
  Gain : Gain  Gain=1.414
  Unit Delay : UnitDelay  SampleTime=-1  HasFrameUpgradeWarning=on
  Unit Delay1 : UnitDelay  SampleTime=-1  HasFrameUpgradeWarning=on
  Unit Delay2 : UnitDelay  SampleTime=-1  HasFrameUpgradeWarning=on
  Out1 : Outport
  wires:
  Divide/1 -> Add5/2
  Unit Delay2/1 -> Add6/1, Add4/2
  Divide2/1 -> Divide1/1, Divide/2
  Add4/1 -> Divide/1
  Unit Delay1/1 -> Add5/1, Add3/1
  Unit Delay/1 -> Add3/2
  Add5/1 -> Out1/1, Divide1/2, Unit Delay1/1
  Add6/1 -> Unit Delay2/1
  Add3/1 -> Gain/1
  Gain/1 -> Add4/1
  Divide1/1 -> Add6/2
  VfMDSP_MotorESpeed_rads/1 -> Divide2/1
  VfMDTM_PwmCycleTime_s/1 -> Divide2/2
  VfMDSP_PhaseUCurVal_A/1 -> Unit Delay/1

== system MDCC_DeadComp/DoCurCtr_sys/MDCC/UdUqCalc_Sys/SelfHeating/Subsystem1/SinCounter_10ms ==
  CNT : Inport
  Add : Sum
  Constant1 : Constant  OutDataTypeStr=uint16
  Constant2 : Constant  Value=0  OutDataTypeStr=uint16
  Delay : Delay  DelayLength=1
  Relational Operator : RelationalOperator  Operator=<=  OutDataTypeStr=boolean  RndMeth=Simplest  InputSameDT=off
  Switch : Switch  Criteria=u2 ~= 0  SaturateOnIntegerOverflow=off  InputSameDT=off
  En : Outport
  wires:
  Add/1 -> Relational Operator/2, Switch/3
  Relational Operator/1 -> Switch/2, En/1  "En"
  Delay/1 -> Add/2
  Constant1/1 -> Add/1
  Constant2/1 -> Switch/1
  Switch/1 -> Delay/1
  CNT/1 -> Relational Operator/1

== system MDCC_DeadComp/DoCurCtr_sys/MDCC/UdUqCalc_Sys/SelfHeating/Subsystem1/Subsystem ==
  VfMDTM_SelfHeatingEAngle_NULL : Inport
  VfMDTM_SelfHeatingUdVal_V_Set : Inport  Port=2
  Enable : EnablePort
  Constant3 : Constant  Value=SinTable12bit_Y
  Direct Lookup Table (n-D)1 : LookupNDDirect  NumberOfTableDimensions=1  TableIsInput=on  Table=[4 5 6]  TableMax=[4096]
  Product : Product
  VfMDTM_SelfHeatingUdVal_V : Outport
  wires:
  Constant3/1 -> Direct Lookup Table (n-D)1/2
  Direct Lookup Table (n-D)1/1 -> Product/1
  VfMDTM_SelfHeatingEAngle_NULL/1 -> Direct Lookup Table (n-D)1/1
  Product/1 -> VfMDTM_SelfHeatingUdVal_V/1
  VfMDTM_SelfHeatingUdVal_V_Set/1 -> Product/2

== system MDCC_DeadComp/DoCurCtr_sys/MDCC/UdUqCalc_Sys/SelfHeating/Subsystem1/Subsystem1 ==
  set : Inport
  rate : Inport  Port=2
  Enable : EnablePort
  Delay : Delay  DelayLength=1
  Relational Operator : RelationalOperator  Operator=<  OutDataTypeStr=boolean  RndMeth=Simplest  InputSameDT=off
  Subsystem1 : Subsystem
  VfMDTM_SelfHeatingUdVal_V_Set : Outport
  VbMDCC_SelfHeatingStop_flg : Outport  Port=2
  wires:
  set/1 -> Subsystem1/1(set)
  Delay/1 -> Subsystem1/3(this_ref)
  Subsystem1/1(VfMDTM_SelfHeatingUdVal_V) -> VfMDTM_SelfHeatingUdVal_V_Set/1, Relational Operator/1, Delay/1
  rate/1 -> Relational Operator/2, Subsystem1/2(rate)
  Relational Operator/1 -> VbMDCC_SelfHeatingStop_flg/1

== system MDCC_DeadComp/DoCurCtr_sys/MDCC/UdUqCalc_Sys/SelfHeating/Subsystem1/Subsystem2 ==
  VfMDTM_SelfHeatingEAngle_NULL : Inport
  VfMDTM_SelfHeatingUdVal_V_Set : Inport  Port=2
  Enable : EnablePort
  Product : Product
  VfMDTM_SelfHeatingUdVal_V : Outport
  wires:
  VfMDTM_SelfHeatingEAngle_NULL/1 -> Product/1
  Product/1 -> VfMDTM_SelfHeatingUdVal_V/1
  VfMDTM_SelfHeatingUdVal_V_Set/1 -> Product/2

== system MDCC_DeadComp/DoCurCtr_sys/MDCC/SVM_Calc/MDSA/SVPWM1/vIntp_PWMFOC_CalSec/CalABC ==
  Bus_Vabc_IN : Inport
  Bus Creator : BusCreator  Inputs=3
  Bus Selector : BusSelector  OutputSignals=Va,Vb,Vc
  CalA : Subsystem
  CalB : Subsystem
  CalC : Subsystem
  Bus_ABC : Outport
  wires:
  Bus_Vabc_IN/1 -> Bus Selector/1
  Bus Selector/1 -> CalA/1(In1)  "<Va>"
  Bus Selector/2 -> CalB/1(In1)  "<Vb>"
  Bus Selector/3 -> CalC/1(In1)  "<Vc>"
  CalB/1(B) -> Bus Creator/2  "B"
  CalC/1(C) -> Bus Creator/3  "C"
  CalA/1(A) -> Bus Creator/1  "A"
  Bus Creator/1 -> Bus_ABC/1

== system MDCC_DeadComp/DoCurCtr_sys/MDCC/SVM_Calc/MDSA/SVPWM1/vIntp_PWMFOC_CalSec/CalSecValue ==
  Bus_ABC_IN : Inport
  Add : Sum  Inputs=+++
  Bus Selector : BusSelector  OutputSignals=A,B,C
  Constant : Constant  Value=2
  Constant1 : Constant  Value=4
  Data Type Conversion : DataTypeConversion  SaturateOnIntegerOverflow=off  RndMeth=Floor
  Data Type Conversion1 : DataTypeConversion  SaturateOnIntegerOverflow=off  RndMeth=Floor
  Data Type Conversion2 : DataTypeConversion  OutDataTypeStr=uint8  SaturateOnIntegerOverflow=off  RndMeth=Floor
  Data Type Conversion3 : DataTypeConversion  OutDataTypeStr=uint8  SaturateOnIntegerOverflow=off  RndMeth=Floor
  Data Type Conversion4 : DataTypeConversion  OutDataTypeStr=uint8  SaturateOnIntegerOverflow=off  RndMeth=Floor
  Lookup_Table : LookupNDDirect  NumberOfTableDimensions=1  Table=[2,2,6,1,4,3,5]  TableDataTypeStr=uint8
      settings: AttributesFormatString=-------------------------------\nTable: %<Table>
  Product : Product
  Product1 : Product
  SecValue : Outport
  N_VALUE : Outport  Port=2
  wires:
  Bus_ABC_IN/1 -> Bus Selector/1
  Constant/1 -> Data Type Conversion/1
  Constant1/1 -> Data Type Conversion1/1
  Data Type Conversion/1 -> Product/2
  Data Type Conversion1/1 -> Product1/2
  Bus Selector/2 -> Product/1  "<B>"
  Bus Selector/3 -> Product1/1  "<C>"
  Bus Selector/1 -> Add/1  "<A>"
  Product/1 -> Data Type Conversion3/1
  Product1/1 -> Data Type Conversion4/1
  Add/1 -> Data Type Conversion2/1
  Data Type Conversion2/1 -> N_VALUE/1, Lookup_Table/1
  Lookup_Table/1 -> SecValue/1
  Data Type Conversion3/1 -> Add/2
  Data Type Conversion4/1 -> Add/3
